simulink model "V2X_Core_SRI_coding_rate_symbol"  (R2023b)
settings: Solver=ode23tb  StartTime=0.0  StopTime=50  MaxStep=1e-2  RelTol=1e-3  AbsTol=1e-3
StopFcn:
  | run('saving.m')
values from neighbouring files (symbols this model uses):
  b = 1.6    [a2024_v2x_matlab_6veh.m]
  m = 2000    [a2024_v2x_matlab_6veh.m]
  mEgo = 1500    [a2024_v2x_matlab_6veh.m]
  Mode = 1    [a2024_v2x_matlab_6veh.m]    (also in v2x_matlab.m; v2x_matlabV2.m; v2x_matlab_6veh.m; v2x_matlab_R.m)
  RefSpeed = 90/3.6    (= 25)    [v2x_matlabV2.m]    (also in v2x_matlab_R.m)
  RelDistThreshold = 300    [v2x_matlabV2.m]    (also in v2x_matlab_R.m)
  s = RandStream("dsfmt19937","Seed",15)    [v2x_matlab.m]
  sampleTime = 0.1    [a2024_v2x_matlab_6veh.m]    (also in v2x_matlab.m; v2x_matlabV2.m; v2x_matlab_6veh.m; v2x_matlab_R.m)
  waypoints = [egoWP(:,2) egoWP(:,1), zeroforwp]    [a2024_v2x_matlab_6veh.m]    (also in misc.m = data.data.ActorSpecifications(1,1).Waypoints(:,[1,2]); v2x_matlab.m = data.data.ActorSpecifications(1,1).Waypoints(:,[1,2]); v2x_matlabV2.m = [5 -1.6 0; v2x_matlab_R.m = [5 -1.6 0)
  ZeroActors = struct(     'ActorID',0,     'Position', [1000 1000 1000],      'Velocity', [0 0 0],      'Roll', 0,      'Pitch', 0,      'Yaw', 0,      'AngularVelocity', [0 0 0])    [v2x_matlabV2.m]    (also in v2x_matlab_R.m)
undefined symbols (not defined in the file or in its folder): Battery, Brakes, Control, DiscIntNeverNeededParam, doppler, Drivetrain, ElectricMotor, Env, FB_flag, Init, SNR_value_list, Vehicle, Wheels
libraries: simulink x45, commofdm x29, commdigbbndam3 x15, commchan3 x14, simulink_extras x13, commcnvcod2 x12, commdigbbndpm3 x11, commblkintrlv2 x10, dspmathops x6, sharedtransform x6, autolibutils x6, autolibsharedcoupling x4
(part 1 of 8)
settings Model: DataDictionary=BEV_ReferenceModel_RWD_Data.sldd  SimulationMode=accelerator  SnapshotBufferSize=50  PacingRate=2  Creator=Fauszt Gábor  LastModifiedBy=user
settings SolverCC: ZeroCrossAlgorithm=Adaptive

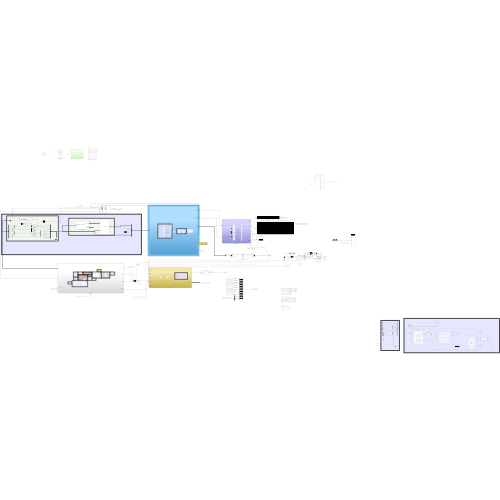
[thumbnail: Simulink's stored preview of the top-level diagram]
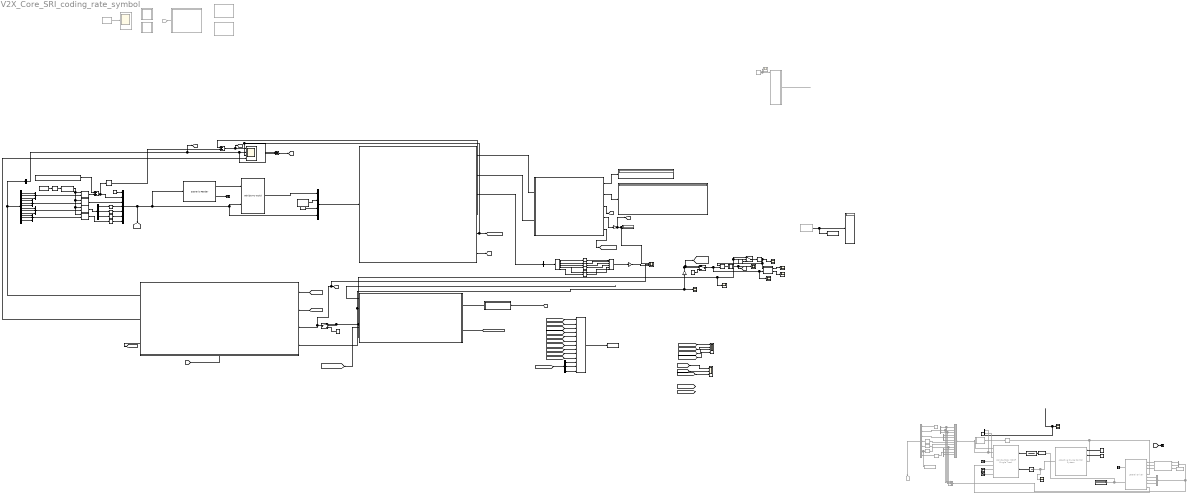
== system V2X_Core_SRI_coding_rate_symbol ==
  note: Scenario Reader
  note: Ego Dynamics
  note: Pack Ego Actor
  note: Pack Ego Actor
  note: V6
  note: V1 Received
  note: V2 Received
  note: V2 Sent
  note: Display block can show only the first 10 columns of a matrix
      | thus, the columns of the 6th vehicle cannot be seen.
  note: V5 Sent
  note: V5
  note: V4
  note: V3 Sent
  note: V3 Received
  note: V1
  note: PDR [%]
  note: V4 Sent
  note: Received correct packets counter
  note: V3
  note: V2
  note: V5 Received
  note: All packets sent counter
  note: V1 Sent
  note: V4 Received
  note: Scenario
  Adaptive Cruise Control System1 : mpcadaslib/Adaptive Cruise Control System  Commented=on  EgoModel=tf(1,[0.5,1,0])  InitialEgoVelocity=20  DefaultSpacing=0  MaxVelocity=20  MinAcceleration=-2  amin_ext=off  MaxAcceleration=4  amax_ext=off  Ts=0.01  PredictionHorizon=3  ControllerBehavior=0.950  suboptimal=off  maxiter=10  datatypeopt=double  optmode=off  trackmode=off
      settings: LibrarySourceBlock=mpclib/Automated Driving/Adaptive Cruise Control System
  Bus Creator : BusCreator  Commented=on  Inputs=4
  Bus Creator1 : BusCreator  Commented=on  Inputs=7  OutDataTypeStr=Bus: Actors  NonVirtualBus=on
      settings: InheritFromInputs=off
  Bus Creator2 : BusCreator  Inputs=4
  Bus Creator3 : BusCreator  Inputs=7  OutDataTypeStr=Bus: Actors  NonVirtualBus=on
      settings: InheritFromInputs=off
  Bus Selector : BusSelector  Commented=on  OutputSignals=InertFrm.Cg.Disp.X,InertFrm.Cg.Disp.Y,InertFrm.Cg.Disp.Z,InertFrm.Cg.Vel.Xdot,InertFrm.Cg.Vel.Ydot,InertFrm.Cg.Vel.Zdot,InertFrm.Cg.Ang.phi,InertFrm.Cg.Ang.theta,InertFrm.Cg.Ang.psi,BdyFrm.Cg.AngVel.p,BdyFrm.Cg.AngVel.q,BdyFrm.Cg.AngVel.r
  Bus Selector1 : BusSelector  Commented=on  OutputSignals=X,Y,psi
  Bus Selector2 : BusSelector  Commented=on  OutputSignals=X,Y
  Bus Selector3 : BusSelector  OutputSignals=InertFrm.Cg.Disp.X,InertFrm.Cg.Disp.Y,InertFrm.Cg.Disp.Z,InertFrm.Cg.Vel.Xdot,InertFrm.Cg.Vel.Ydot,InertFrm.Cg.Vel.Zdot,InertFrm.Cg.Ang.phi,InertFrm.Cg.Ang.theta,InertFrm.Cg.Ang.psi,BdyFrm.Cg.AngVel.p,BdyFrm.Cg.AngVel.q,BdyFrm.Cg.AngVel.r
  Bus Selector4 : BusSelector  OutputSignals=BdyFrm.Cg.Vel.xdot
  Bus Selector8 : BusSelector  OutputSignals=ActorRxPower
  Calculate PDR : Subsystem
  Channel : Subsystem  Commented=on
  Compare To Constant1 : simulink/Logic and Bit Operations/Compare To Constant  relop=>=  const=-69  OutDataTypeStr=boolean
  Compare To Constant2 : simulink/Logic and Bit Operations/Compare To Constant  relop=>=  const=-68  OutDataTypeStr=boolean
  Compare To Constant3 : simulink/Logic and Bit Operations/Compare To Constant  relop=>=  const=-82  OutDataTypeStr=boolean
  Compare To Constant4 : simulink/Logic and Bit Operations/Compare To Constant  relop=>=  const=-80  OutDataTypeStr=boolean
  Compare To Constant5 : simulink/Logic and Bit Operations/Compare To Constant  relop=>=  const=-69  OutDataTypeStr=boolean
  Compare To Constant6 : simulink/Logic and Bit Operations/Compare To Constant  relop=>=  const=-82  OutDataTypeStr=boolean
  Constant : Constant  Value=1e-1
  Constant1 : Constant  Value=200
  Constant10 : Constant  Commented=on  Value=waypoints
  Constant11 : Constant  Commented=on  SampleTime=-1
  Constant12 : Constant  Value=20  VectorParams1D=off  SampleTime=sampleTime
  Constant13 : Constant  Value=1.4  VectorParams1D=off  SampleTime=sampleTime
  Constant2 : Constant  Value=[pi 0 0]
  Constant3 : Constant  Value=[-Vehicle.CG.LongDistRearAxle 0 0]
  Constant4 : Constant  Value=RelDistThreshold
  Constant7 : Constant  SampleTime=-1
  Counter Limited1 : simulink/Sources/Counter Limited  Commented=on  uplimit=0  tsamp=0.01
  DSRC : Subsystem
  Data Type Conversion : DataTypeConversion  SaturateOnIntegerOverflow=off  RndMeth=Floor
  DelayMessage1 : Subsystem  mask{delay=0, sampleTime=sampleTime}
      mask prompts: delay "Delay in sec"; sampleTime "MessageInSampleTime"
  Demux : Demux  Outputs=3
  Demux1 : Demux  Outputs=3
  Display{,1,14..16} (5 alike) : Display
  Divide : Product  Inputs=*/
  Ego trajectory : MATLAB Function  Commented=on  TreatAsAtomicUnit=on
  From1 : From  Commented=on
  Gain : Gain  Gain=100
  Gain1 : Gain  Gain=100
  Gain3 : Gain  Gain=-1
  Goto : Goto  Commented=on
  Integrator : Integrator
  Lateral Driver : vehdynlibdriver/Lateral Driver  Commented=on  extSteerOvr=off  extSteerHld=off  extSteerZero=off  steerOut=off  cntrlTypeLat=Stanley  coordMode=SAE J670 (Z-down)  angUnits=rad  tau=0.1  L=3  vecPose=off  dynamMode=on  PositionGainF=2.5  PositionGainR=2.5  YawRateGain=.2  DelayGain=.2  a=a  b=b  m=mEgo  Cy_f=Cy_f  Cy_r=70933  I=4013  Ksteer=18  theta=45*pi/180  aMode=2
  Low pass filter : TransferFcn  Denominator=[0.001 1]
  MATLAB Function : MATLAB Function  TreatAsAtomicUnit=on
  MATLAB Function1 : MATLAB Function  TreatAsAtomicUnit=on
  MATLAB Function2 : MATLAB Function  Commented=on  TreatAsAtomicUnit=on
  MATLAB Function3 : MATLAB Function  Commented=on  TreatAsAtomicUnit=on
  MATLAB Function6 : MATLAB Function  Commented=on  TreatAsAtomicUnit=on
  MATLAB Function8 : MATLAB Function  TreatAsAtomicUnit=on
  MatrixMultiply{,1..3} (4 alike) : Product  Multiplication=Matrix(*)
  Memory : Memory  Commented=on  InitialCondition=1
  MsgSendTrigger : simulink_extras/Flip Flops/Clock  period=0.1
  Mux : Mux  Commented=on  Inputs=3
  Mux1 : Mux  Commented=on  Inputs=3
  Mux2 : Mux  Commented=on  Inputs=3
  Mux{3..6} (4 alike) : Mux  Inputs=3
  Perception : Subsystem
  Pilot Port : Subsystem  ReferencedSubsystem=Pilot_Port
  Radians to Degrees{,1..3} (4 alike) : simulink_extras/Transformations/Radians to Degrees  Commented=on
  Radians to Degrees{4..7} (4 alike) : simulink_extras/Transformations/Radians to Degrees
  Rotation Angles to Direction Cosine Matrix : sharedtransform/Rotation Angles to Direction Cosine Matrix  rotationOrder=ZYX  aMode=aMode
  SISO Fading Channel : commchan3/SISO Fading Channel  Commented=through  InheritSampleRate=off  SampleRate=5.9e9  PathDelays=0  AveragePathGains=0  NormalizePathGains=on  FadingDistribution=Rayleigh  KFactor=3  DirectPathDopplerShift=0  DirectPathInitialPhase=0  MaximumDopplerShift=0.001  DopplerSpectrum=doppler('Jakes')  RandomStream=mt19937ar with seed  Seed=73  PathGainsOutputPort=off  ChannelFilterDelayOutputPort=off  SimulateUsing=Interpreted execution  Visualization=Off  PathsForDopplerDisplay=1  SamplesToDisplay=25%
  Scenario Reader1 : drivingscenarioandsensors/Scenario Reader  ScenarioSource=From file  ScenarioFileName=C:\Users\user\Desktop\Fauszt_Gabor_matlab_v2x\Driving scenarios\TEST_1000_stationary.mat  ScenarioVariableName=scenario  OutputCoordinateSystem=Vehicle coordinates  EgoVehicleSource=Input port  EgoVehicleActorID=1  OrientVehiclesOnRoad=off  OutputEgoVehiclePose=on  OutputEgoVehicleState=off  SampleTime=sampleTime  LaneBoundaryOutput=All lane boundaries  LaneBoundaryDistance=0:0.5:9.5  LaneBoundaryLocation=Center of lane markings  BusNameSource=Auto  BusName=ActorsAll  BusNumActorsSource=Scenario  BusNumActors=100  BusName2Source=Auto  BusName2=BusLaneBoundaries  BusNumLaneBoundariesSource=Scenario  BusNumLaneBoundaries=10  BusName3Source=Auto  BusName3=BusEgoActor  BusName4Source=Auto  BusName4=BusEgoState  ShowCoordinateLabels=on  SimulateUsing=Interpreted execution
  Scope : Scope  NumInputPorts=3
  Scope{1..3,5..9,14} (9 alike) : Scope
  Scope10 : Scope  NumInputPorts=4
  Scope11 : Scope  NumInputPorts=4
  Scope12 : Scope  NumInputPorts=3
  Scope13 : Scope  Commented=on
  Scope4 : Scope  Commented=on
  Selector : Selector  InputPortWidth=3  IndexOptions=Index vector (dialog)  Indices=1  OutputSizes=1
  Selector1 : Selector  InputPortWidth=3  IndexOptions=Index vector (dialog)  Indices=[3 2 1]  OutputSizes=1
  Subsystem1 : Subsystem  Commented=on
  Subsystem2 : Subsystem  Commented=on
  Subtract : Sum
  Subtract1 : Sum  Inputs=+-
  Subtract2 : Sum  Inputs=+-
  Switch : Switch  SaturateOnIntegerOverflow=off  InputSameDT=off
  Switch1 : Switch  Criteria=u2 > Threshold  Threshold=1  SaturateOnIntegerOverflow=off  InputSameDT=off
  Switch2 : Switch  Criteria=u2 > Threshold  SaturateOnIntegerOverflow=off  InputSameDT=off
  Terminator{,7..11} (6 alike) : Terminator
  To Workspace1 : ToWorkspace  VariableName=Channelout  SampleTime=-1
  To Workspace2 : ToWorkspace  Commented=on  VariableName=yaw  SampleTime=-1
  To Workspace3 : ToWorkspace  VariableName=SNR0_stat_aeb  SaveFormat=Structure With Time  SampleTime=-1
  Variant Sink1 : VariantSink
  Variant Source1 : VariantSource
  Vector Concatenate : Concatenate
  Vector Concatenate1 : Concatenate  NumInputs=13
  Vehicle 2 : Subsystem  Commented=on
  Vehicle 3 : Subsystem  Commented=on
  Vehicle Body 3DOF Single Track1 : autolibshared/Vehicle Body 3DOF Single Track  Commented=on  trackMode=Single (bicycle)  inputMode=External longitudinal velocity  frontSteerMode=on  rearSteerMode=off  windMode=off  muMode=off  extFMode=off  extMMode=off  htchFMode=off  htchMMode=off  extXo=off  extpsio=off  extxdoto=off  extro=off  extYo=off  extTamb=off  extydoto=off  aMode=2  NF=nrWheelsFr  NR=nrWheelsRe  m=mEgo  a=a  b=b  h=h  dh=1  hh=0.2  X_o=waypoints(1,1)  xdot_o=0  CalphaMode=off  sigmaMode=on  d=0  hl=0  w=[1.4,1.4]  Cy_f=Cy_f  Cy_r=Cy_r  sigma_f=sigma_f  sigma_r=sigma_r  alpha_f_brk=[-.1 .1]  Cy_f_data=[-9e3 9e3]  alpha_r_brk=[-.1 .1]  Cy_r_data=[-9e3 9e3]  Y_o=waypoints(1,2)  ydot_o=0  Izz=Izz  psi_o=deg2rad(waypoints(1,3))  r_o=deg2rad(waypoints(1,3))  Af=2  Cd=.3  Cl=.1  Cpm=.1  beta_w=[0 0.01:0.01:0.3]  Cs=[0 0.01:0.01:0.3]  Cym=[0 1e-6:0.01:0.3]  Pabs=101325  Tair=273  g=9.81  mu=1  xdot_tol=.01  Fznom=5000  Fxtire_sat=7e4  Fytire_sat=7e4  longOff=0  latOff=0  vertOff=0  wrapAng=off
  Vehicle To World : drivingscenarioandsensors/Vehicle To World  BusNameSource=Auto  BusName=ActorsaAll  SimulateUsing=Interpreted execution
  VehicleDynamic : Subsystem
      settings: PortSchema="{\"entries\":[{\"content\":{\"sides\":[{\"content\":{\"connectorIds\":[\"In1\",\"In2\",\"In3\",\"In4\"]},\"type\":\"ConnectorPlacement.EquallySpacedRectSide\",\"uuid\":\"5cebcc0e-9aab-459f-b090-1519655ce47f\"},{\"content\":{\"connectorIds\":[\"Out1\",\"Out2\",\"Out3\"],\"side\":\"RIGHT\"},\"type\":\"ConnectorPlacement.EquallySpacedRectSide\",\"uuid\":\"f32df9e5-ba46-47a7-861c-9e33fbf56710\"},{\"content\":{\"side\":\"TOP\"},\"type\":\"ConnectorPlacement.EquallySpacedRectSide\",\"uuid\":\"4ea7047d-6198-49e7-925a-91d5ec867f77\"},{\"content\":{\"connectorIds\":[\"In5\"],\"side\":\"BOTTOM\"},\"type\":\"ConnectorPlacement.EquallySpacedRectSide\",\"uuid\":\"3b7d66be-9692-4aa1-9991-122eb4adbaf4\"}]},\"type\":\"ConnectorPlacement.EquallySpacedConnector\",\"uuid\":\"14d79c81-525e-43ad-a5bc-0ffd345a9605\"}],\"packageUris\":[\"http://schema.mathworks.com/mf0/Connector/R2020b\"],\"version\":\"1.0\"}"
  wires:
  From1/1 -> Channel/1(EgoData)
  Scenario Reader1/2 -> Terminator/1
  MATLAB Function3/1(Dist) -> Scope4/1
  Scenario Reader1/1 -> Vehicle To World/1
  Vehicle To World/1 -> Bus Creator2/1  "Actors"
  SISO Fading Channel/1 -> To Workspace1/1, Display/1
  Radians to Degrees2/1 -> Bus Creator1/5  "Pitch"
  Adaptive Cruise Control System1/1 -> Scope7/1, Integrator/1  "Acceleration of ego"
  Ego trajectory/3(YawRef) -> Lateral Driver/3
  Vehicle Body 3DOF Single Track1/6 -> Terminator9/1
  Bus Selector/5 -> Mux2/2  "<Ydot>"
  Vector Concatenate/1 -> Scope6/1
  Bus Selector2/1 -> Ego trajectory/1(EgoFdbX)  "<X>"
  Bus Selector1/3 -> Lateral Driver/8  "<psi>"
  [B] -> Terminator7/1
  Memory/1 -> Lateral Driver/5, Adaptive Cruise Control System1/3
  Radians to Degrees/1 -> Bus Creator1/7  "AngularVelocity"
  Vehicle Body 3DOF Single Track1/5 -> Lateral Driver/9  "r"
  Bus Selector1/2 -> Lateral Driver/7  "<Y>"
  MATLAB Function6/1(y) -> Memory/1
  Constant13/1 -> Adaptive Cruise Control System1/2
  Lateral Driver/2 -> Data Type Conversion/1, Display15/1
  Integrator/1 -> Vehicle Body 3DOF Single Track1/2
  Constant12/1 -> Adaptive Cruise Control System1/1
  Radians to Degrees1/1 -> Bus Creator1/4  "Roll"
  Vehicle Body 3DOF Single Track1/7 -> Terminator11/1
  Low pass filter/1 -> Vehicle Body 3DOF Single Track1/1
  Ego trajectory/1(LongRef) -> Lateral Driver/1
  Constant10/1 -> Ego trajectory/3(waypoints)
  Vehicle Body 3DOF Single Track1/2 -> Vector Concatenate/1, MATLAB Function6/1(xdotin)  "Longitudinal velocity of ego"
  Bus Selector/7 -> Radians to Degrees1/1  "<phi>"
  Vehicle Body 3DOF Single Track1/3 -> Vector Concatenate/2
  Data Type Conversion/1 -> Low pass filter/1
  Bus Selector1/1 -> Lateral Driver/6  "<X>"
  Bus Creator1/1 -> Goto/1  "Actors"
  Vehicle Body 3DOF Single Track1/1 -> Bus Selector/1
  Bus Selector/11 -> Mux/2  "<q>"
  Bus Selector/12 -> Mux/3  "<r>"
  Bus Selector2/2 -> Ego trajectory/2(EgoFdbY)  "<Y>"
  Bus Selector/9 -> Radians to Degrees3/1, Bus Creator/4  "<psi>"
  Bus Selector/3 -> Mux1/3, Bus Creator/3  "<Z>"
  Bus Creator/1 -> Bus Selector2/1, Bus Selector1/1
  Bus Selector/1 -> Bus Creator/1, Mux1/1  "<X>"
  Ego trajectory/2(LatRef) -> Lateral Driver/2
  Radians to Degrees3/1 -> To Workspace2/1, Bus Creator1/6  "Yaw"
  Bus Selector/2 -> Bus Creator/2, Mux1/2  "<Y>"
  Mux2/1 -> Bus Creator1/3  "Velocity"
  Lateral Driver/1 -> Terminator10/1
  Bus Selector/10 -> Mux/1  "<p>"
  Mux/1 -> Radians to Degrees/1
  Vehicle Body 3DOF Single Track1/4 -> Terminator8/1
  Bus Selector/8 -> Radians to Degrees2/1  "<theta>"
  Bus Selector/6 -> Mux2/3  "<Zdot>"
  Mux1/1 -> Bus Creator1/2  "Position"
  Constant11/1 -> Bus Creator1/1  "ActorID"
  Bus Selector/4 -> Mux2/1  "<Xdot>"
  Bus Selector3/11 -> Mux3/2  "<q>"
  Constant7/1 -> Bus Creator3/1  "ActorID"
  Bus Selector3/4 -> Mux5/1  "<Xdot>"
  Bus Selector3/1 -> Mux4/1  "<X>"
  Bus Selector3/6 -> Mux5/3  "<Zdot>"
  Bus Selector3/10 -> Mux3/1  "<p>"
  Bus Selector3/2 -> Mux4/2  "<Y>"
  Radians to Degrees6/1 -> Bus Creator3/5  "Pitch"
  Radians to Degrees5/1 -> Bus Creator3/4  "Roll"
  Radians to Degrees4/1 -> Bus Creator3/7  "AngularVelocity"
  Bus Selector3/3 -> Mux4/3  "<Z>"
  Bus Selector3/5 -> Mux5/2  "<Ydot>"
  Radians to Degrees7/1 -> Bus Creator3/6  "Yaw"
  Bus Selector3/12 -> Mux3/3  "<r>"
  Bus Creator3/1 -> Scenario Reader1/1, Bus Creator2/4, Vehicle To World/2, [EgoData]  "Ego"
  Calculate PDR/2(Sent and Received vectors side by side for comparison) -> Display14/1
  Calculate PDR/1(PDR) -> Display16/1
  VehicleDynamic/1(Out1) -> Bus Selector4/1, Bus Selector3/1
  Constant2/1 -> Selector1/1
  Selector1/1 -> Rotation Angles to Direction Cosine Matrix/1
  Bus Selector3/7 -> Mux6/1  "<phi>"
  Bus Selector3/8 -> Mux6/2  "<theta>"
  Bus Selector3/9 -> Mux6/3  "<psi>"
  Rotation Angles to Direction Cosine Matrix/1 -> MatrixMultiply1/1, MatrixMultiply2/1, MatrixMultiply3/1, MatrixMultiply/1
  Mux4/1 -> MatrixMultiply/2  "Position"
  Mux5/1 -> MatrixMultiply1/2  "Velocity"
  Mux6/1 -> MatrixMultiply2/2
  Mux3/1 -> MatrixMultiply3/2
  MatrixMultiply3/1 -> Radians to Degrees4/1
  MatrixMultiply2/1 -> Demux/1
  Demux/1 -> Radians to Degrees5/1
  Demux/2 -> Radians to Degrees6/1
  Demux/3 -> Radians to Degrees7/1
  MatrixMultiply1/1 -> Bus Creator3/3
  MatrixMultiply/1 -> Subtract/2
  Constant3/1 -> Subtract/1
  Subtract/1 -> Selector/1, Bus Creator3/2
  Selector/1 -> Subtract1/2
  Bus Selector4/1 -> [Ego_Velocity], Subtract2/2, Scope11/2  "<xdot>"
  Subtract1/1 -> [RelativeDistance_GT], Scope11/1  "RelativeDistance_GT"
  Calculate PDR/3(Rx) -> [Rx]
  [Rx] -> DelayMessage1/1(ActorDataToSend)
  MsgSendTrigger/1 -> Bus Creator2/3  "Trigger"
  Pilot Port/1 -> Bus Creator2/2  "Pilot"
  ? -> MATLAB Function2/2(Actor1)  "<Actor1>"
  MATLAB Function2/1(y) -> ?
  Counter Limited1/1 -> Scope13/1, MATLAB Function2/1(Control)  "Control"
  Calculate PDR/4(PDR/sec) -> Gain/1
  Gain/1 -> [PDR], Scope/1, Display1/1  "PDR%"
  VehicleDynamic/2(sri_val) -> Scope11/4  "Sri_val"
  [RelativeSpeed] -> VehicleDynamic/1(u)
  [PDR] -> VehicleDynamic/2(PDR)
  Bus Selector8/1 -> Variant Sink1/1  "<ActorRxPower>"
  Gain1/1 -> Scope/3  "Receive"
  Perception/1(RelativeDist1) -> ?
  DelayMessage1/1(ActorDataReceived) -> Perception/1(Rx)  "Rx"
  [EgoData] -> Perception/2(EgoData)
  Perception/4(RelativeSpeed) -> [RelativeSpeed]
  Bus Creator2/1 -> DSRC/1(In13)
  DSRC/1(SentPacket) -> Calculate PDR/1(Sent packets (Actors bus from Scenario Reader))
  DSRC/3(Actor1) -> Bus Selector8/1
  DSRC/4(PosX) -> Subtract1/1
  DSRC/5(RV_Speed) -> [RV_Velocity], Scope11/3, Subtract2/1  "RV_Speed"
  DSRC/2(ReceivedPacket) -> Calculate PDR/2(Received packets (Matrix from the processed data by ego))
  Variant Sink1/4 -> Compare To Constant4/1
  Compare To Constant3/1 -> Variant Source1/3
  Variant Sink1/2 -> Compare To Constant2/1
  Compare To Constant1/1 -> Variant Source1/1
  Compare To Constant2/1 -> Variant Source1/2
  Compare To Constant4/1 -> Variant Source1/4
  Variant Sink1/1 -> Compare To Constant1/1
  Variant Sink1/3 -> Compare To Constant3/1
  Variant Source1/1 -> Gain1/1
  Switch/1 -> Scope9/1, MATLAB Function/2(Rel_Vel), Divide/2
  Constant/1 -> Switch/3
  Divide/1 -> MATLAB Function1/1(u)
  Perception/2(RelativeVelocity) -> VehicleDynamic/4(RelativeVelocity), Scope2/1, Gain3/1
  Perception/5(TTC_Dist) -> Switch2/2, Switch2/1, Scope14/1, Switch1/1, Switch1/2
  Gain3/1 -> [RelativeVelocity_Perc], Switch/1, Switch/2
  MATLAB Function/1(TTC) -> Scope3/1
  MATLAB Function/2(FB_Flag) -> Scope5/1
  Constant1/1 -> Switch1/3
  Switch1/1 -> MATLAB Function8/1(u)
  MATLAB Function8/1(RelDist) -> Scope8/1, Divide/1, MATLAB Function/1(Rel_Dist)  "RelativeDist"
  [RelativeDistance_GT] -> Scope10/1  "RelDist_GT"
  [RelativeDistance_Perc] -> Scope10/2  "RelDist_Perc"
  [PDR] -> Scope10/3  "PDR"
  VehicleDynamic/3(Acc from Control) -> [AccfromControl]
  [AccfromControl] -> Scope12/1  "Acceleration of Control"
  [Ego_Velocity] -> Scope12/2  "Ego Velocity"
  [RelativeDistance_Perc] -> Scope12/3  "RelDist_Perc"
  DSRC/6(SNR) -> [SNR]
  [SNR] -> Scope10/4  "SNR"
  Subtract2/1 -> [RelativeVelocity_GT]  "RelativeVelocity_GT"
  [RelativeDistance_GT] -> Vector Concatenate1/1  "RelDist_GT"
  [RelativeDistance_Perc] -> Vector Concatenate1/2  "RelDist_Perc"
  [RelativeVelocity_GT] -> Vector Concatenate1/3  "RelVel_GT"
  [RelativeVelocity_Perc] -> Vector Concatenate1/4  "RelVel_Perc"
  [Ego_Velocity] -> Vector Concatenate1/5  "Ego Velocity"
  [RV_Velocity] -> Vector Concatenate1/6  "RV_Speed"
  [PDR] -> Vector Concatenate1/7  "PDR"
  [SNR] -> Vector Concatenate1/8  "SNR"
  [TTC] -> Vector Concatenate1/9  "TTC"
  [AccfromControl] -> Vector Concatenate1/10  "Accel of Control"
  Vector Concatenate1/1 -> To Workspace3/1
  Variant Sink1/5 -> Compare To Constant5/1
  Compare To Constant5/1 -> Variant Source1/5
  Variant Sink1/6 -> Compare To Constant6/1
  Compare To Constant6/1 -> Variant Source1/6
  Switch2/1 -> Scope/2, [RelativeDistance_Perc], VehicleDynamic/3(RelDist)
  Constant4/1 -> Switch2/3
  Calculate PDR/5(Packets) -> [Packets]
  [Packets] -> Demux1/1  "Packets"
  Demux1/1 -> Vector Concatenate1/11  "PDR for full"
  Demux1/2 -> Vector Concatenate1/12  "Received Packets"
  Demux1/3 -> Vector Concatenate1/13  "Sent Packets"
  [TTC] -> VehicleDynamic/5(TTC)
  MATLAB Function1/1(RelDist) -> [TTC], Scope1/1  "RelativeDist"

== system V2X_Core_SRI_coding_rate_symbol/Calculate PDR ==
  Sent packets (Actors bus from Scenario Reader) : Inport
  Received packets (Matrix from the processed data by ego) : Inport  Port=2
  Bus Creator : BusCreator  Inputs=12
  Bus Selector : BusSelector  OutputSignals=PDR V1,PDR V2,PDR V3,PDR V4,PDR V5,PDR V6
  Bus Selector1 : BusSelector  OutputSignals=Vectors V1,Vectors V2,Vectors V3,Vectors V4,Vectors V5,Vectors V6
  Constant1 : Constant  Value=2
  Constant2 : Constant  Value=3
  Constant3 : Constant  Value=4
  Constant4 : Constant  Value=5
  Constant5 : Constant
  Constant6 : Constant  Value=6
  Matrix Concatenate : Concatenate  NumInputs=6  Mode=Multidimensional array  ConcatenateDimension=2
  Matrix Concatenate2 : Concatenate  NumInputs=6  Mode=Multidimensional array  ConcatenateDimension=2
  PDR V1 : Subsystem
  PDR V2 : Subsystem
  PDR V3 : Subsystem
  PDR V4 : Subsystem
  PDR V5 : Subsystem
  PDR V6 : Subsystem
  PDR : Outport
  Sent and Received vectors side by side for comparison : Outport  Port=2
  Rx : Outport  Port=3
  PDR/sec : Outport  Port=4
  Packets : Outport  Port=5
  wires:
  Bus Selector1/6 -> Matrix Concatenate/6  "<Vectors V6>"
  Bus Creator/1 -> Bus Selector/1, Bus Selector1/1
  Bus Selector1/3 -> Matrix Concatenate/3  "<Vectors V3>"
  PDR V1/2(Vectors output) -> Bus Creator/2  "Vectors V1"
  Sent packets (Actors bus from Scenario Reader)/1 -> PDR V6/1(Sent packet), PDR V5/1(Sent packet), PDR V4/1(Sent packet), PDR V3/1(Sent packet), PDR V2/1(Sent packet), PDR V1/1(Sent packet)
  Received packets (Matrix from the processed data by ego)/1 -> PDR V6/2(Received packets), PDR V5/2(Received packets), PDR V4/2(Received packets), PDR V3/2(Received packets), PDR V2/2(Received packets), PDR V1/2(Received packets)
  PDR V5/1(PDR1) -> Bus Creator/9  "PDR V5"
  Matrix Concatenate/1 -> Sent and Received vectors side by side for comparison/1  "Sent and Received vectors side by side"
  Constant1/1 -> PDR V2/3(Vehicle ID)
  PDR V3/2(Vectors output) -> Bus Creator/6  "Vectors V3"
  Bus Selector/1 -> Matrix Concatenate2/1  "<PDR V1>"
  Bus Selector1/4 -> Matrix Concatenate/4  "<Vectors V4>"
  Constant4/1 -> PDR V5/3(Vehicle ID)
  Bus Selector/4 -> Matrix Concatenate2/4  "<PDR V4>"
  Bus Selector1/5 -> Matrix Concatenate/5  "<Vectors V5>"
  Bus Selector1/1 -> Matrix Concatenate/1  "<Vectors V1>"
  Bus Selector1/2 -> Matrix Concatenate/2  "<Vectors V2>"
  PDR V6/2(Vectors output) -> Bus Creator/12  "Vectors V6"
  Bus Selector/5 -> Matrix Concatenate2/5  "<PDR V5>"
  Constant3/1 -> PDR V4/3(Vehicle ID)
  PDR V2/2(Vectors output) -> Bus Creator/4  "Vectors V2"
  Constant6/1 -> PDR V6/3(Vehicle ID)
  Bus Selector/3 -> Matrix Concatenate2/3  "<PDR V3>"
  Bus Selector/6 -> Matrix Concatenate2/6  "<PDR V6>"
  Bus Selector/2 -> Matrix Concatenate2/2  "<PDR V2>"
  PDR V1/1(PDR1) -> Packets/1, Bus Creator/1  "PDR V1"
  Constant5/1 -> PDR V1/3(Vehicle ID)
  Constant2/1 -> PDR V3/3(Vehicle ID)
  PDR V5/2(Vectors output) -> Bus Creator/10  "Vectors V5"
  PDR V2/1(PDR2) -> Bus Creator/3  "PDR V2"
  PDR V3/1(PDR3) -> Bus Creator/5  "PDR V3"
  PDR V4/2(Vectors output) -> Bus Creator/8  "Vectors V4"
  PDR V4/1(PDR1) -> Bus Creator/7  "PDR V4"
  PDR V6/1(PDR1) -> Bus Creator/11  "PDR V6"
  Matrix Concatenate2/1 -> PDR/1  "PDR"
  PDR V1/3(Rx) -> Rx/1
  PDR V1/4(PDR/sec) -> PDR/sec/1

== system V2X_Core_SRI_coding_rate_symbol/Channel ==
  EgoData : Inport
  AWGN Channel : commchan3/AWGN Channel  LegacyMode=off  NoiseMethod="Signal to noise ratio  (SNR)"  noiseMode="Signal to noise ratio  (SNR)"  EbNo=10  EsNo=10  SNR=60  BitsPerSymbol=1  SignalPower=1  SamplesPerSymbol=1  SymbolPeriod=1  VarianceSource=Parameter  Variance=1  RandomStream=Global stream  Seed=67  SimulateUsing=Interpreted execution
  Constant : Constant  Value=ZeroActors  OutDataTypeStr=Bus: Actors  SampleTime=sampleTime
  Constant1 : Constant  Commented=on  Value=randn(10)+55  SampleTime=sampleTime
  Entity Multicast : EntityMulticast  InputPortMessageModes=m  MulticastTag=B
  Entity Multicast1 : EntityMulticast  InputPortMessageModes=m  MulticastTag=B
  Entity Multicast2 : EntityMulticast  InputPortMessageModes=m  MulticastTag=B
  MATLAB Function1 : MATLAB Function  TreatAsAtomicUnit=on
  MATLAB Function4 : MATLAB Function  TreatAsAtomicUnit=on
  MATLAB Function9 : MATLAB Function  TreatAsAtomicUnit=on
  Multicast Receive Queue : Queue  OutputPortMessageModes=m  EntityArrivalSource=Multicast
  Receive : Receive  InputPortMessageModes=m  UseInternalQueue=off  QueueOverwriting=on  QueueLength=1  QueueType=LIFO
  Scope : Scope
  Send : Send  OutputPortMessageModes=m
  Send1 : Send  OutputPortMessageModes=m
  Send2 : Send  OutputPortMessageModes=m
  Terminator : Terminator
  wires:
  Multicast Receive Queue/1 -> Receive/1
  AWGN Channel/1 -> MATLAB Function1/1(ActorsIn)
  Receive/1 -> AWGN Channel/1
  MATLAB Function1/1(Actors) -> MATLAB Function9/2(Actors)
  MATLAB Function1/2(Positions) -> MATLAB Function9/3(Positions)  "Positions"
  Constant/1 -> MATLAB Function9/4(ZeroActors)
  MATLAB Function9/4(PSR) -> MATLAB Function4/1(PSR)
  MATLAB Function9/3(ThresholdActor) -> Send/1
  MATLAB Function9/2(InterferingActor) -> Send2/1
  MATLAB Function9/1(LeadActor) -> Send1/1
  EgoData/1 -> MATLAB Function9/1(Ego), MATLAB Function1/2(Ego)
  Constant1/1 -> ?
  MATLAB Function1/3(Distances) -> Terminator/1  "Distances"
  MATLAB Function4/1(CBR) -> Scope/1
  Send1/1 -> Entity Multicast2/1
  Send2/1 -> Entity Multicast1/1
  Send/1 -> Entity Multicast/1

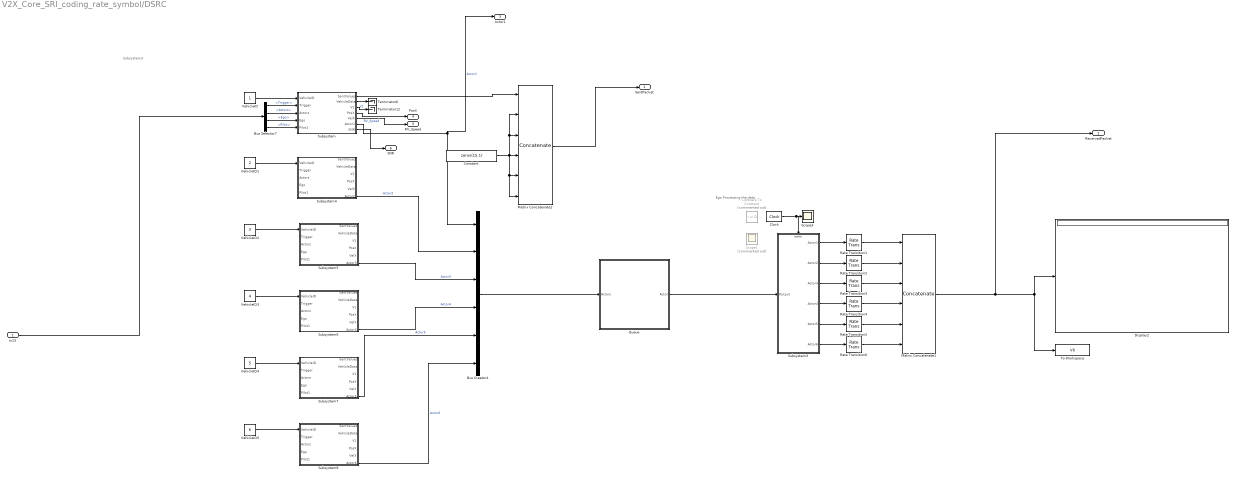
== system V2X_Core_SRI_coding_rate_symbol/DSRC ==
  note: Ego Processing the data
  note: Subsystem3
  In13 : Inport
  Bus Creator4 : BusCreator  Inputs=6
  Bus Selector7 : BusSelector  OutputSignals=Trigger,Actors,Ego,Pilot
  Clock : simulink_extras/Flip Flops/Clock  period=0.01
  Compare To Constant : simulink/Logic and Bit Operations/Compare To Constant  Commented=on  relop=~=  const=0  OutDataTypeStr=uint8
  Constant : Constant  Value=zeros(15,1)
  Display2 : Display
  Matrix Concatenate1 : Concatenate  NumInputs=6  Mode=Multidimensional array  ConcatenateDimension=2
  Matrix Concatenate2 : Concatenate  NumInputs=6  Mode=Multidimensional array  ConcatenateDimension=2
  Queue : Subsystem
  Rate Transition{1..6} (6 alike) : RateTransition  OutPortSampleTime=sampleTime/10
  Scope1 : Scope  Commented=on
  Scope3 : Scope
  Subsystem : Subsystem
  Subsystem3 : Subsystem
  Subsystem4 : Subsystem
  Subsystem5 : Subsystem
  Subsystem6 : Subsystem
  Subsystem7 : Subsystem
  Subsystem8 : Subsystem
  Terminator12 : Terminator
  Terminator6 : Terminator
  To Workspace : ToWorkspace  VariableName=V6  SampleTime=-1
  VehicleID : Constant
  VehicleID1 : Constant  Value=2
  VehicleID2 : Constant  Value=3
  VehicleID3 : Constant  Value=4
  VehicleID4 : Constant  Value=5
  VehicleID5 : Constant  Value=6
  SentPacket : Outport
  ReceivedPacket : Outport  Port=2
  Actor1 : Outport  Port=3
  PosX : Outport  Port=4
  RV_Speed : Outport  Port=5
  SNR : Outport  Port=6
  wires:
  Rate Transition6/1 -> Matrix Concatenate1/6
  VehicleID4/1 -> Subsystem7/1(VehicleID)
  Subsystem3/2(Actor2) -> Rate Transition2/1
  Constant/1 -> Matrix Concatenate2/6, Matrix Concatenate2/5, Matrix Concatenate2/2, Matrix Concatenate2/3, Matrix Concatenate2/4
  Rate Transition2/1 -> Matrix Concatenate1/2
  Subsystem3/1(Actor1) -> Rate Transition1/1
  Matrix Concatenate2/1 -> SentPacket/1
  Rate Transition3/1 -> Matrix Concatenate1/3
  Bus Selector7/2 -> Subsystem/3(Actors)  "<Actors>"
  Subsystem/3(V1) -> Terminator12/1  "V1"
  Bus Selector7/3 -> Subsystem/4(Ego)  "<Ego>"
  Subsystem5/6(Actor3) -> Bus Creator4/3  "Actor3"
  Subsystem/5(VelX) -> RV_Speed/1  "RV_Speed"
  Subsystem3/6(Actor6) -> Rate Transition6/1
  Rate Transition5/1 -> Matrix Concatenate1/5
  Subsystem3/5(Actor5) -> Rate Transition5/1
  VehicleID/1 -> Subsystem/1(VehicleID)
  Bus Selector7/1 -> Subsystem/2(Trigger)  "<Trigger>"
  Bus Selector7/4 -> Subsystem/5(Pilot1)  "<Pilot>"
  Subsystem/6(Actor1) -> Actor1/1, Bus Creator4/1  "Actor1"
  Subsystem/2(VehicleData) -> Terminator6/1
  Subsystem3/3(Actor3) -> Rate Transition3/1
  Subsystem3/4(Actor4) -> Rate Transition4/1
  Subsystem6/6(Actor4) -> Bus Creator4/4  "Actor4"
  Clock/1 -> Scope3/1, Subsystem3/Enable
  Subsystem8/6(Actor6) -> Bus Creator4/6  "Actor6"
  Matrix Concatenate1/1 -> Display2/1, To Workspace/1, ReceivedPacket/1
  Rate Transition1/1 -> Matrix Concatenate1/1
  Rate Transition4/1 -> Matrix Concatenate1/4
  Subsystem7/6(Actor5) -> Bus Creator4/5  "Actor5"
  In13/1 -> Bus Selector7/1
  Subsystem4/6(Actor2) -> Bus Creator4/2  "Actor2"
  Subsystem/1(SentValues) -> Matrix Concatenate2/1
  VehicleID3/1 -> Subsystem6/1(VehicleID)
  VehicleID5/1 -> Subsystem8/1(VehicleID)
  VehicleID2/1 -> Subsystem5/1(VehicleID)
  VehicleID1/1 -> Subsystem4/1(VehicleID)
  Subsystem/4(PosX) -> PosX/1
  Queue/1(Actor) -> Subsystem3/1(Output)
  Bus Creator4/1 -> Queue/1(Actors)
  Subsystem/7(SNR) -> SNR/1

== system V2X_Core_SRI_coding_rate_symbol/DelayMessage1 ==
  ActorDataToSend : Inport
  Clock : simulink_extras/Flip Flops/Clock  period=sampleTime
  Product : Product
  Queue : Queue  InputPortMessageModes=m  OutputPortMessageModes=m  OverwriteOldest=on  Capacity=ceil(delay/sampleTime)+1
  Send : Send  OutputPortMessageModes=m
  Step : Step  Time=delay  SampleTime=0
  Subsystem : Subsystem
  ActorDataReceived : Outport
  wires:
  ActorDataToSend/1 -> Send/1
  Subsystem/1(Out) -> ActorDataReceived/1
  Product/1 -> Subsystem/Trigger
  Queue/1 -> Subsystem/1(Queue)
  Clock/1 -> Product/2
  Send/1 -> Queue/1
  Step/1 -> Product/1

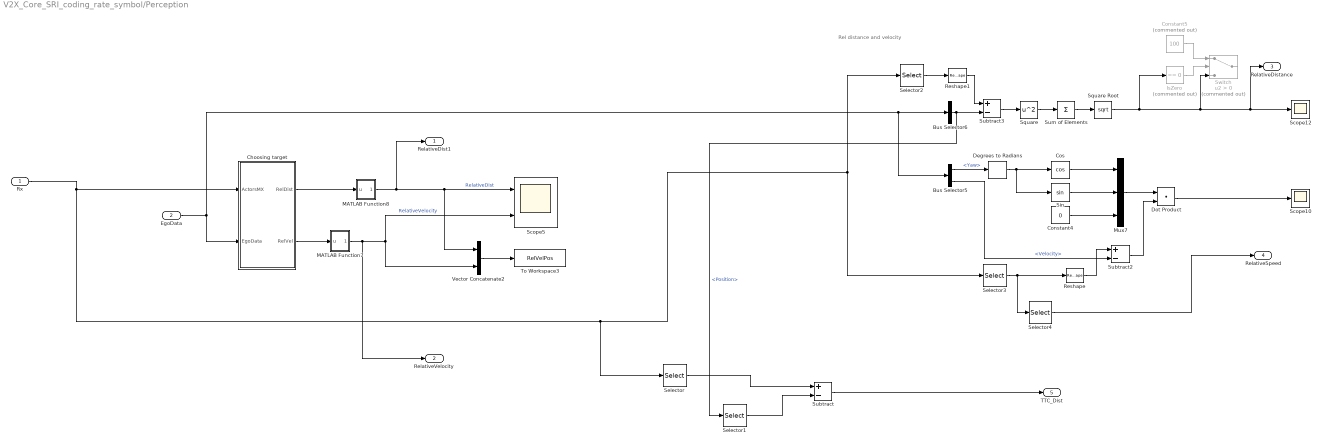
== system V2X_Core_SRI_coding_rate_symbol/Perception ==
  note: Rel distance and velocity
  Rx : Inport
  EgoData : Inport  Port=2
  Bus Selector5 : BusSelector  OutputSignals=Yaw,Velocity
  Bus Selector6 : BusSelector  OutputSignals=Position
  "Choosing target " : MATLAB Function  TreatAsAtomicUnit=on
  Constant4 : Constant  Value=0
  Constant5 : Constant  Commented=on  Value=100
  Cos : Trigonometry  Operator=cos
  Degrees to Radians : simulink_extras/Transformations/Degrees to Radians
  Dot Product : DotProduct  OutDataTypeStr=Inherit: Inherit via internal rule
  IsZero : simulink/Logic and Bit Operations/Compare To Zero  Commented=on  relop===  OutDataTypeStr=boolean
      settings: LibrarySourceBlock=|
      | simulink/Quick Insert/Logic and Bit
      | Operations/IsZero
  MATLAB Function7 : MATLAB Function  TreatAsAtomicUnit=on
  MATLAB Function8 : MATLAB Function  TreatAsAtomicUnit=on
  Mux7 : Mux  Inputs=3
  Reshape : Reshape  OutputDimensionality=Row vector (2-D)
  Reshape1 : Reshape  OutputDimensionality=Row vector (2-D)
  Scope10 : Scope
  Scope12 : Scope
  Scope5 : Scope  NumInputPorts=2
  Selector : Selector  InputPortWidth=15  IndexOptions=Index vector (dialog)  Indices=[4]  OutputSizes=1
  Selector1 : Selector  InputPortWidth=3  IndexOptions=Index vector (dialog)  Indices=[1]  OutputSizes=1
  Selector2 : Selector  InputPortWidth=15  IndexOptions=Index vector (dialog)  Indices=[4:6]  OutputSizes=1
  Selector3 : Selector  InputPortWidth=15  IndexOptions=Index vector (dialog)  Indices=[7:9]  OutputSizes=1
  Selector4 : Selector  InputPortWidth=3  IndexOptions=Index vector (dialog)  Indices=1  OutputSizes=1
  Sin : Trigonometry
  Square : Math  Operator=square
  Square Root : Sqrt
  Subtract : Sum  Inputs=+-
  Subtract2 : Sum  Inputs=+-
  Subtract3 : Sum  Inputs=+-
  Sum of Elements : Sum  Inputs=+
  Switch : Switch  Commented=on  Criteria=u2 > Threshold  SaturateOnIntegerOverflow=off  InputSameDT=off
  To Workspace3 : ToWorkspace  VariableName=RelVelPos  SampleTime=-1
  Vector Concatenate2 : Concatenate
  RelativeDist1 : Outport
  RelativeVelocity : Outport  Port=2
  RelativeDistance : Outport  Port=3
  RelativeSpeed : Outport  Port=4
  TTC_Dist : Outport  Port=5
  wires:
  Rx/1 -> Selector/1, Selector2/1, Selector3/1, "Choosing target "/1(ActorsMX)
  Square/1 -> Sum of Elements/1
  Subtract2/1 -> Dot Product/2
  Selector2/1 -> Reshape1/1
  Dot Product/1 -> Scope10/1
  Sum of Elements/1 -> Square Root/1
  Cos/1 -> Mux7/1
  Bus Selector6/1 -> Selector1/1, Subtract3/2  "<Position>"
  MATLAB Function7/1(RelVel) -> RelativeVelocity/1, Vector Concatenate2/2, Scope5/2  "RelativeVelocity"
  Mux7/1 -> Dot Product/1
  IsZero/1 -> Switch/2
  Degrees to Radians/1 -> Sin/1, Cos/1
  Vector Concatenate2/1 -> To Workspace3/1
  Subtract3/1 -> Square/1
  Selector3/1 -> Reshape/1, Selector4/1
  Sin/1 -> Mux7/2
  Bus Selector5/2 -> Subtract2/2  "<Velocity>"
  Reshape1/1 -> Subtract3/1
  MATLAB Function8/1(RelDist) -> Vector Concatenate2/1, Scope5/1, RelativeDist1/1  "RelativeDist"
  Constant5/1 -> Switch/1
  Reshape/1 -> Subtract2/1
  Constant4/1 -> Mux7/3
  EgoData/1 -> Bus Selector5/1, Bus Selector6/1, "Choosing target "/2(EgoData)
  Bus Selector5/1 -> Degrees to Radians/1  "<Yaw>"
  "Choosing target "/1(RelDist) -> MATLAB Function8/1(u)
  "Choosing target "/2(RelVel) -> MATLAB Function7/1(u)
  Selector4/1 -> RelativeSpeed/1
  Square Root/1 -> IsZero/1, Switch/3, RelativeDistance/1, Scope12/1
  Selector/1 -> Subtract/1
  Selector1/1 -> Subtract/2
  Subtract/1 -> TTC_Dist/1

== system V2X_Core_SRI_coding_rate_symbol/Subsystem1 ==
  VehicleID : Inport
  Trigger : Inport  Port=2
  busActors3Test1 : Inport  Port=3
  Pilot : Inport  Port=4
  Actors : Inport  Port=5
  Constant2 : Constant  Value=[zeros(19,1)']  SampleTime=-1
  Entity Multicast1 : EntityMulticast  InputPortMessageModes=m
  Integer to Bit Converter2 : simulink/Logic and Bit Operations/Integer to Bit Converter  nbits=16  signedInputValues=Signed  bitOrder=MSB first  outDtype=boolean
  MATLAB Function1 : MATLAB Function  TreatAsAtomicUnit=on
  OFDM Modulator : commofdm/OFDM Modulator  StatePerturbationForJacobian=1.0e-05  FFTLength=64  NumGuardBandCarriers=[0;0]  InsertDCNull=on  PilotInputPort=on  PilotCarrierIndices=[12; 26; 40; 54]  CyclicPrefixLength=32  Windowing=off  WindowLength=16  OversamplingFactor=3  NumSymbols=1  NumTransmitAntennas=1  SimulateUsing=Interpreted execution
  Rectangular QAM Modulator Baseband2 : commdigbbndam3/Rectangular QAM Modulator Baseband  M=2^6  InType=Bit  Enc=Binary  Mapping=[0:15]  PowType=Average Power  MinDist=2  AvgPow=P_Signal  PeakPow=1  Ph=0  outDtype=double  outWordLen=16  outUDDataType=sfix(16)  outFracLenMode=Best precision  outFracLen=15  outDataTypeStr=double  outLastDataTypeStr=double
      settings: LibrarySourceBlock=|
      | commhdldigbbndam/Rectangular QAM
      | Modulator
      | Baseband
  Send1 : Send  OutputPortMessageModes=m
  Vector Concatenate : Concatenate
  VehicleData : Outport
  V2 : Outport  Port=2
  wires:
  MATLAB Function1/3(counter) -> V2/1
  MATLAB Function1/2(VehicleData) -> VehicleData/1
  Pilot/1 -> OFDM Modulator/2
  VehicleID/1 -> MATLAB Function1/2(VehicleID)
  busActors3Test1/1 -> MATLAB Function1/1(busActors3Test1)
  Trigger/1 -> MATLAB Function1/Trigger
  Integer to Bit Converter2/1 -> Rectangular QAM Modulator Baseband2/1
  OFDM Modulator/1 -> Send1/1  "OFDM modulated"
  Actors/1 -> MATLAB Function1/3(EgoData)
  Constant2/1 -> Vector Concatenate/2
  Rectangular QAM Modulator Baseband2/1 -> Vector Concatenate/1
  Send1/1 -> Entity Multicast1/1
  Vector Concatenate/1 -> OFDM Modulator/1  "After QAM Mod"
  MATLAB Function1/1(Actor) -> Integer to Bit Converter2/1

== system V2X_Core_SRI_coding_rate_symbol/Subsystem2 ==
  VehicleID : Inport
  Trigger : Inport  Port=2
  busActors3Test1 : Inport  Port=3
  Pilot : Inport  Port=4
  Actors : Inport  Port=5
  Constant2 : Constant  Value=[zeros(19,1)']  SampleTime=-1
  Display : Display
  Entity Multicast1 : EntityMulticast  InputPortMessageModes=m
  Integer to Bit Converter2 : simulink/Logic and Bit Operations/Integer to Bit Converter  nbits=16  signedInputValues=Signed  bitOrder=MSB first  outDtype=boolean
  MATLAB Function1 : MATLAB Function  TreatAsAtomicUnit=on
  OFDM Modulator : commofdm/OFDM Modulator  StatePerturbationForJacobian=1.0e-05  FFTLength=64  NumGuardBandCarriers=[0;0]  InsertDCNull=on  PilotInputPort=on  PilotCarrierIndices=[12; 26; 40; 54]  CyclicPrefixLength=32  Windowing=off  WindowLength=16  OversamplingFactor=3  NumSymbols=1  NumTransmitAntennas=1  SimulateUsing=Interpreted execution
  Rectangular QAM Modulator Baseband2 : commdigbbndam3/Rectangular QAM Modulator Baseband  M=2^6  InType=Bit  Enc=Binary  Mapping=[0:15]  PowType=Average Power  MinDist=2  AvgPow=P_Signal  PeakPow=1  Ph=0  outDtype=double  outWordLen=16  outUDDataType=sfix(16)  outFracLenMode=Best precision  outFracLen=15  outDataTypeStr=double  outLastDataTypeStr=double
      settings: LibrarySourceBlock=|
      | commhdldigbbndam/Rectangular QAM
      | Modulator
      | Baseband
  Send1 : Send  OutputPortMessageModes=m
  To Workspace : ToWorkspace  VariableName=v3  SampleTime=-1
  Vector Concatenate : Concatenate
  VehicleData : Outport
  V3 : Outport  Port=2
  wires:
  MATLAB Function1/1(Actor) -> To Workspace/1, Display/1, Integer to Bit Converter2/1
  Vector Concatenate/1 -> OFDM Modulator/1  "After QAM Mod"
  Send1/1 -> Entity Multicast1/1
  Rectangular QAM Modulator Baseband2/1 -> Vector Concatenate/1
  Constant2/1 -> Vector Concatenate/2
  Actors/1 -> MATLAB Function1/3(EgoData)
  OFDM Modulator/1 -> Send1/1  "OFDM modulated"
  Integer to Bit Converter2/1 -> Rectangular QAM Modulator Baseband2/1
  Trigger/1 -> MATLAB Function1/Trigger
  busActors3Test1/1 -> MATLAB Function1/1(busActors3Test1)
  VehicleID/1 -> MATLAB Function1/2(VehicleID)
  Pilot/1 -> OFDM Modulator/2
  MATLAB Function1/2(VehicleData) -> VehicleData/1
  MATLAB Function1/3(counter) -> V3/1

== system V2X_Core_SRI_coding_rate_symbol/Vehicle 2 ==
  trigger : Inport
  VehicleID : Inport  Port=2
  Pilot : Inport  Port=3
  busActors3Test1 : Inport  Port=4
  Constant2 : Constant  Value=[zeros(19,1)']  SampleTime=-1
  Entity Multicast1 : EntityMulticast  InputPortMessageModes=m
  Integer to Bit Converter1 : simulink/Logic and Bit Operations/Integer to Bit Converter  nbits=16  signedInputValues=Signed  bitOrder=MSB first  outDtype=boolean
  MATLAB Function1 : MATLAB Function  TreatAsAtomicUnit=on
  OFDM Modulator1 : commofdm/OFDM Modulator  StatePerturbationForJacobian=1.0e-05  FFTLength=64  NumGuardBandCarriers=[0;0]  InsertDCNull=on  PilotInputPort=on  PilotCarrierIndices=[12; 26; 40; 54]  CyclicPrefixLength=32  Windowing=off  WindowLength=16  OversamplingFactor=3  NumSymbols=1  NumTransmitAntennas=1  SimulateUsing=Interpreted execution
  Rectangular QAM Modulator Baseband1 : commdigbbndam3/Rectangular QAM Modulator Baseband  M=2^6  InType=Bit  Enc=Binary  Mapping=[0:15]  PowType=Average Power  MinDist=2  AvgPow=P_Signal  PeakPow=1  Ph=0  outDtype=double  outWordLen=16  outUDDataType=sfix(16)  outFracLenMode=Best precision  outFracLen=15  outDataTypeStr=double  outLastDataTypeStr=double
      settings: LibrarySourceBlock=|
      | commhdldigbbndam/Rectangular QAM
      | Modulator
      | Baseband
  Send1 : Send  OutputPortMessageModes=m
  Vector Concatenate1 : Concatenate
  wires:
  busActors3Test1/1 -> MATLAB Function1/1(busActors3Test1)
  Rectangular QAM Modulator Baseband1/1 -> Vector Concatenate1/1
  Constant2/1 -> Vector Concatenate1/2
  Send1/1 -> Entity Multicast1/1
  Integer to Bit Converter1/1 -> Rectangular QAM Modulator Baseband1/1
  Vector Concatenate1/1 -> OFDM Modulator1/1  "After QAM Mod"
  OFDM Modulator1/1 -> Send1/1  "OFDM modulated"
  MATLAB Function1/1(intVector) -> Integer to Bit Converter1/1
  trigger/1 -> MATLAB Function1/Trigger
  VehicleID/1 -> MATLAB Function1/2(VehicleID)
  Pilot/1 -> OFDM Modulator1/2

== system V2X_Core_SRI_coding_rate_symbol/Vehicle 3 ==
  trigger : Inport
  busActors3Test1 : Inport  Port=2
  Pilot : Inport  Port=3
  VehicleID : Inport  Port=4
  Constant3 : Constant  Value=[zeros(19,1)']  SampleTime=-1
  Entity Multicast2 : EntityMulticast  InputPortMessageModes=m
  Integer to Bit Converter3 : simulink/Logic and Bit Operations/Integer to Bit Converter  nbits=16  signedInputValues=Signed  bitOrder=MSB first  outDtype=boolean
  MATLAB Function2 : MATLAB Function  TreatAsAtomicUnit=on
  OFDM Modulator2 : commofdm/OFDM Modulator  StatePerturbationForJacobian=1.0e-05  FFTLength=64  NumGuardBandCarriers=[0;0]  InsertDCNull=on  PilotInputPort=on  PilotCarrierIndices=[12; 26; 40; 54]  CyclicPrefixLength=32  Windowing=off  WindowLength=16  OversamplingFactor=3  NumSymbols=1  NumTransmitAntennas=1  SimulateUsing=Interpreted execution
  Rectangular QAM Modulator Baseband3 : commdigbbndam3/Rectangular QAM Modulator Baseband  M=2^6  InType=Bit  Enc=Binary  Mapping=[0:15]  PowType=Average Power  MinDist=2  AvgPow=P_Signal  PeakPow=1  Ph=0  outDtype=double  outWordLen=16  outUDDataType=sfix(16)  outFracLenMode=Best precision  outFracLen=15  outDataTypeStr=double  outLastDataTypeStr=double
      settings: LibrarySourceBlock=|
      | commhdldigbbndam/Rectangular QAM
      | Modulator
      | Baseband
  Send2 : Send  OutputPortMessageModes=m
  Vector Concatenate2 : Concatenate
  wires:
  MATLAB Function2/1(intVector) -> Integer to Bit Converter3/1
  OFDM Modulator2/1 -> Send2/1  "OFDM modulated"
  busActors3Test1/1 -> MATLAB Function2/1(busActors3Test1)
  Vector Concatenate2/1 -> OFDM Modulator2/1  "After QAM Mod"
  Send2/1 -> Entity Multicast2/1
  Integer to Bit Converter3/1 -> Rectangular QAM Modulator Baseband3/1
  Rectangular QAM Modulator Baseband3/1 -> Vector Concatenate2/1
  Pilot/1 -> OFDM Modulator2/2
  Constant3/1 -> Vector Concatenate2/2
  VehicleID/1 -> MATLAB Function2/2(VehicleID)
  trigger/1 -> MATLAB Function2/Trigger
